simulink model "frac_cap"  (R2024a)
settings: Solver=FixedStepAuto  StartTime=0.0  StopTime=15  FixedStep=0.0001  RelTol=1e-3
undefined symbols (not defined in the file): A, alpha, DIM, G, X0
libraries: cstblocks x2
settings Model: Creator=dawid  LastModifiedBy=dawid

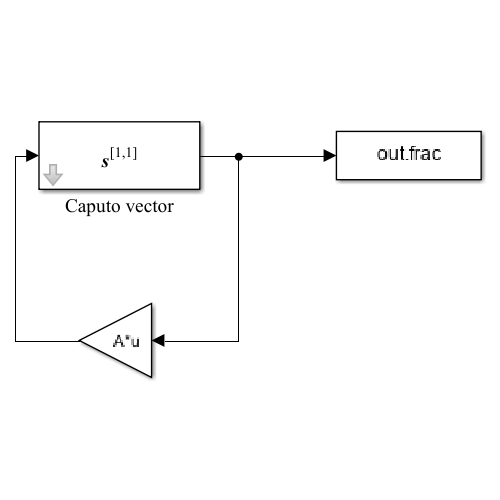
[thumbnail: Simulink's stored preview of the top-level diagram]
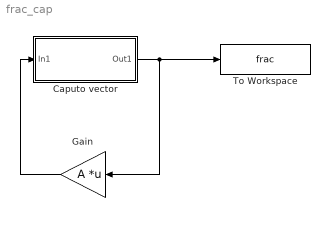
== system frac_cap ==
  Caputo vector : Subsystem  mask{gam=alpha, ww=[1e-4 1e4], N=11, M=DIM, x0=X0}
      mask prompts: gam "Derivative order gamma"; ww "Frequency range [wb,wh]"; N "Approximation order N"; M "Dimension M"; x0 "Initial condition x0"
      mask init:
      | wb=ww(1); wh=ww(2); stri=[];
      | if length(gam)==1, gam=gam*ones(M,1); end
      | for i=1:M
      |     G(i,1)=ousta_fod(1-gam(i),N,wb,wh); stri=[stri,num2str(gam(i)),','];
      | end
      | str=['{\bf{\its}}^{[' stri(1:end-1) ']}'];
      | svec2sl(gam);
      mask Display: disp(str,'texmode','on')
  Gain : Gain  Gain=A  Multiplication=Matrix(K*u)
  To Workspace : ToWorkspace  VariableName=frac  SaveFormat=Structure With Time  SampleTime=-1
  wires:
  Gain/1 -> Caputo vector/1(In1)
  Caputo vector/1(Out1) -> To Workspace/1, Gain/1

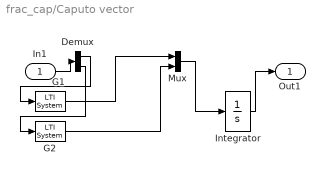
== system frac_cap/Caputo vector ==
  In1 : Inport
  Demux : Demux  Outputs=2
  G1 : cstblocks/LTI System  sys=G(1)  IC=[]  PadeOrder=0
  G2 : cstblocks/LTI System  sys=G(2)  IC=[]  PadeOrder=0
  Integrator : Integrator  InitialCondition=x0
  Mux : Mux  Inputs=2
  Out1 : Outport
  wires:
  Demux/1 -> G1/1
  G1/1 -> Mux/1
  Demux/2 -> G2/1
  G2/1 -> Mux/2
  Integrator/1 -> Out1/1
  Mux/1 -> Integrator/1
  In1/1 -> Demux/1
